simulink model "InversePendulum"  (R2023a)
settings: Solver=VariableStepAuto  StartTime=0.0  StopTime=10.0  RelTol=1e-3
settings Model: Creator=Diman18  LastModifiedBy=Diman18

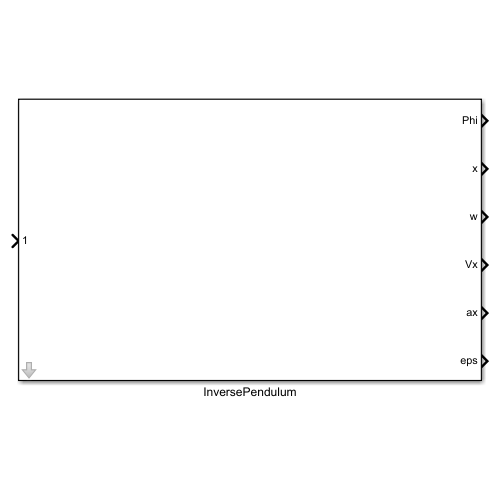
[thumbnail: Simulink's stored preview of the top-level diagram]
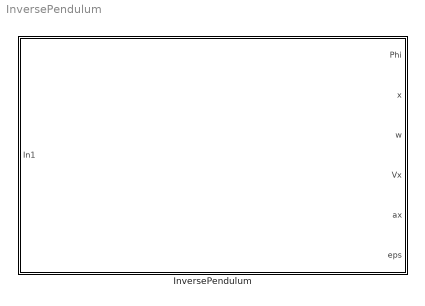
== system InversePendulum ==
  InversePendulum : Subsystem  mask{M_ctergnya=0.1, Lc=1, M_telegi=0.2, g=9.8}

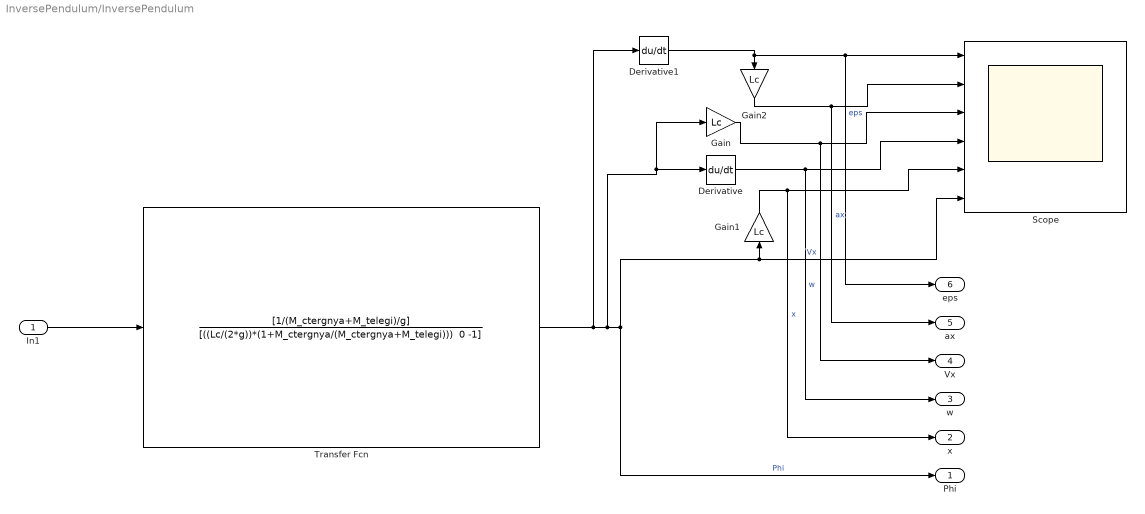
== system InversePendulum/InversePendulum ==
  In1 : Inport
  Derivative : Derivative
  Derivative1 : Derivative
  Gain : Gain  Gain=Lc
  Gain1 : Gain  Gain=Lc
  Gain2 : Gain  Gain=Lc
  Scope : Scope  NumInputPorts=6
  Transfer Fcn : TransferFcn  Numerator=[1/(M_ctergnya+M_telegi)/g]  Denominator="[((Lc/(2*g))*(1+M_ctergnya/(M_ctergnya+M_telegi)))  0 -1]"
  Phi : Outport
  x : Outport  Port=2
  w : Outport  Port=3
  Vx : Outport  Port=4
  ax : Outport  Port=5
  eps : Outport  Port=6
  wires:
  In1/1 -> Transfer Fcn/1
  Transfer Fcn/1 -> Derivative1/1, Gain/1, Derivative/1, Scope/6, Gain1/1, Phi/1  "Phi"
  Derivative/1 -> w/1, Scope/4  "w"
  Derivative1/1 -> Gain2/1, eps/1, Scope/1  "eps"
  Gain/1 -> Vx/1, Scope/3  "Vx"
  Gain1/1 -> x/1, Scope/5  "x"
  Gain2/1 -> ax/1, Scope/2  "ax"
